simulink model "counter_unit_testing"  (R2019b)
settings: Solver=FixedStepDiscrete  StartTime=0.0  StopTime=10.0  FixedStep=1  MaxStep=1  RelTol=1e-3
undefined symbols (not defined in the file): sigbuilder_block
settings Model: Creator=chiragg  LastModifiedBy=chiragg

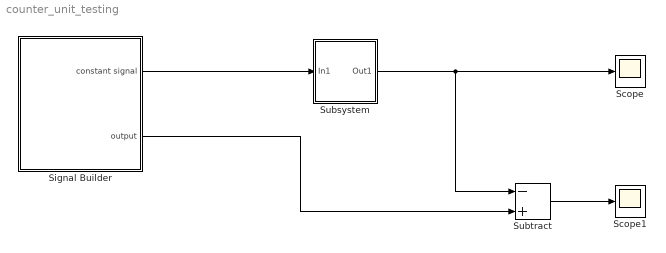
== system counter_unit_testing ==
  Scope : Scope
  Scope1 : Scope
  Signal Builder : Subsystem  Tag=STV Subsys  LoadFcn=sigbuilder_block('load');  StartFcn=sigbuilder_block('start');  StopFcn=sigbuilder_block('stop');  ClipboardFcn=sigbuilder_block('clipboard');  mask(Sigbuilder block){tuvar=[0:10]}
      mask help: Simulink:masks:SigbuilderBlock_MD
      mask init:
      | if ~strcmp(get_param(bdroot(gcbh),'SimulationStatus'),'stopped') tuvar = sigbuilder_block('maskInit'); end
      settings: CopyFcn=sigbuilder_block('copy');  DeleteFcn=sigbuilder_block('delete');  ModelCloseFcn=sigbuilder_block('modelClose');  PreSaveFcn=sigbuilder_block('preSave');  PauseFcn=sigbuilder_block('pause');  ContinueFcn=sigbuilder_block('continue');  NameChangeFcn=sigbuilder_block('namechange');  OpenFcn=sigbuilder_block('open',[6 30 1428 681.75 ]);  CloseFcn=sigbuilder_block('close');
      mask Display: plot(0, 0, 100, 100,[2, 2, 32, 32, 2], [68, 8, 8, 68, 68],[32, 2], [38, 38], [32, 19, 2],[53, 60, 44], [32, 17, 17, 2],[16, 16, 31, 31]);txt = getActiveGroup(gcbh);text(2, 100, txt,'verticalAlignment', 'top');
  Subsystem : Subsystem
  Subtract : Sum  Inputs=-+
  wires:
  Subsystem/1(Out1) -> Subtract/1, Scope/1
  Subtract/1 -> Scope1/1
  Signal Builder/1(constant signal) -> Subsystem/1(In1)
  Signal Builder/2(output) -> Subtract/2

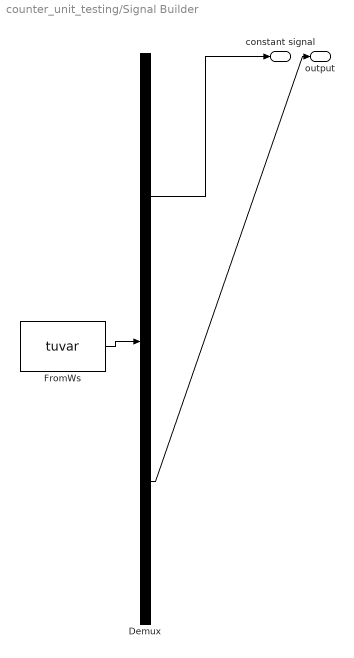
== system counter_unit_testing/Signal Builder ==
  Demux : Demux  Tag=STV Demux  Outputs=2
  FromWs : FromWorkspace  Tag=STV FromWs  VariableName=tuvar  SampleTime=0
      SigBuilderData=|
      | common.afterFinalStr = 'Extrapolate'
      | common.sampleTime = 0
      | dataSet.timeRange = [0 10]
      | dataSet.name = 'Group 1'
      | sbobj.Groups.Name = 'Group 1'
      | sbobj.Groups.Signals(1).Name = 'constant signal'
      | sbobj.Groups.Signals(1).XData = [0 10]
      | sbobj.Groups.Signals(1).YData = [1 1]
      | sbobj.Groups.Signals(2).Name = 'output'
      | sbobj.Groups.Signals(2).XData = [0 0.5 1 1 1.5 2 2 3 3 4 4 5 5 6 6 7 7 8 8 9 9 10]
      | sbobj.Groups.Signals(2).YData = [1 1 1 2 2 2 3 3 4 4 5 5 6 6 7 7 8 8 9 9 10 10]
  constant signal : Outport  Tag=STV Outport
  output : Outport  Tag=STV Outport  Port=2
  wires:
  Demux/1 -> constant signal/1
  FromWs/1 -> Demux/1
  Demux/2 -> output/1

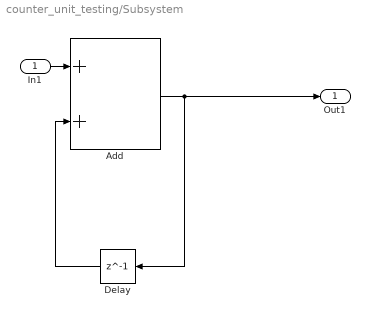
== system counter_unit_testing/Subsystem ==
  In1 : Inport
  Add : Sum
  Delay : Delay  DelayLength=1
  Out1 : Outport
  wires:
  Add/1 -> Out1/1, Delay/1
  Delay/1 -> Add/2
  In1/1 -> Add/1
